simulink model "Day6playingwithscopeandsources"  (R2023b)
settings: Solver=VariableStepAuto  StartTime=0.0  StopTime=40.0  RelTol=1e-3
libraries: simulink x3
settings Model: Creator=ray  LastModifiedBy=ray

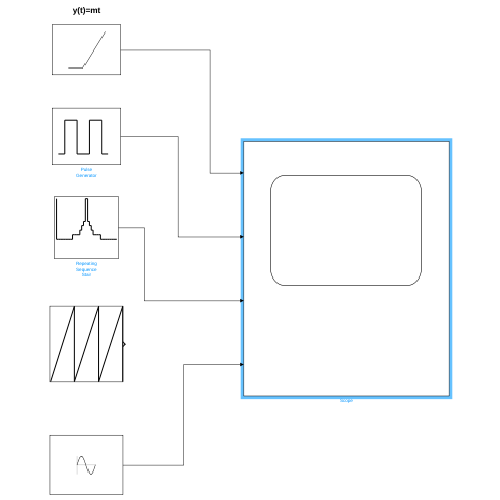
[thumbnail: Simulink's stored preview of the top-level diagram]
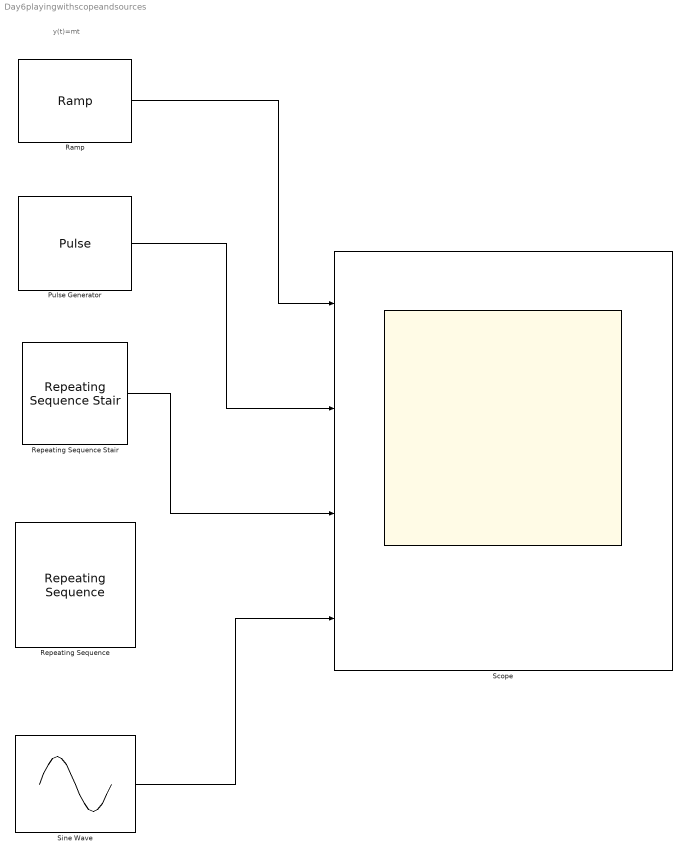
== system Day6playingwithscopeandsources ==
  note: y(t)=mt
  Pulse Generator : DiscretePulseGenerator  PulseType=Time based  Amplitude=5  Period=20  PulseWidth=20
  Ramp : simulink/Sources/Ramp  slope=1  start=0  InitialOutput=0
  Repeating Sequence : simulink/Sources/Repeating Sequence  rep_seq_t=[0 5]  rep_seq_y=[0 8]
  Repeating Sequence Stair : simulink/Sources/Repeating Sequence Stair  OutValues=[1 1 1 1 1 1 1 1 1 2 2 2 2 3 4 5 10 5 4 3 2 2 2 2 1 1 1 1 1 1 1 1 1 ].'  tsamp=-1  OutMin=[]  OutMax=[]  OutDataTypeStr=double  OutputDataTypeScalingMode=double  OutDataType=fixdt(0,8)  ConRadixGroup=Best Precision: Vector-wise  OutScaling=2^-12
  Scope : Scope  NumInputPorts=4
  Sine Wave : Sin  Amplitude=5  Frequency=0.2  SampleTime=0
  wires:
  Sine Wave/1 -> Scope/4
  Ramp/1 -> Scope/1
  Pulse Generator/1 -> Scope/2
  Repeating Sequence Stair/1 -> Scope/3
